simulink library "SUB_ECU_L4_MABX_HW_Interface_PTC_1571"  (R2018a)
settings: Solver=VariableStepAuto  StartTime=0.0  StopTime=10.0  RelTol=1e-3
PostLoadFcn:
  | , if any(exist('dsrtsu_mdlpostloadfcn', 'file') == [2, 3, 6]), try dsrtsu_mdlpostloadfcn('Execute', bdroot); catch fprintf('Error in PostLoadFcn (dsrtsu_mdlpostloadfcn) for model "%s":\n %s\n', bdroot, lasterr); end, end,
undefined symbols (not defined in the file or in its folder): CANR_PROPB_REAX_3_13_CHANNEL_APV, CANR_PROPB_REAX_4_13_CHANNEL_APV, CANR_PROPB_XPR_1_50_CHANNEL_APV, ENUM_CAN_RX_T, ENUM_CAN_TX_T, ENUM_REAX_OPERATION_MODE_T, ENUM_SIGNAL_HEALTH_T, ENUM_XBR_CONTROL_MODE_T, ENUM_XBR_EBI_MODE_T, ENUM_XBR_PASS_THROUGH_ACTIVE_T, ENUM_XBR_PRIORITY_T, ENUM_XPR_INHIBIT_PARK_MANUAL_T, ENUM_XPR_INHIBIT_UNPARK_MANUAL_T, ENUM_XPR_PARK_MANUAL_T, ENUM_XPR_UNPARK_MANUAL_T, IGNITION_RELAY_OVERRIDE_APV, INVERTER_RELAY_OVERRIDE_APV, MABX_RELAY_OVERRIDE_APV, PROPB_REAX_1_E4_DES_POS_SIG_SRC_APV, PROPB_REAX_1_E4_DESIRED_OPMODE_APV, PROPB_REAX_1_E4_DESIRED_POSITION_APV, ptc_matlab_lib, SENSOR_RELAY_OVERRIDE_APV, sfi, sfp
libraries: PTC_MBDS_LIB x163, rtican x81, simulink x41, EmE_MBD_Blockset x35, rti1401lib_dio_type4 x8, simulink_need_slupdate x7, $bdroot x5, rti1401lib_adc_type4 x2, rti1401lib_aio_type1 x1, rtitasklib x1
(part 5 of 27)

== system SUB_ECU_L4_MABX_HW_Interface_PTC_1571/DIGITAL_out/Shift Control ==
  In : Inport
  Bus Creator1 : BusCreator  Inputs=1
  Bus Selector : BusSelector  OutputSignals=INPUTS.DIO_Bus.ShiftControlDC
  Bus Selector1 : BusSelector  OutputSignals=INPUTS.CAN.ETC2_03.SPN524_TransSelectedGear,INPUTS.CAN.ETC2_03.SPN523_TransCurrentGear
  Compare To Zero : simulink/Logic and Bit Operations/Compare To Zero  relop===  OutDataTypeStr=boolean
  Compare To Zero1 : simulink/Logic and Bit Operations/Compare To Zero  relop===  OutDataTypeStr=boolean
  Constant : Constant  Value=.4
  Constant1 : Constant  Value=0.5
  Constant2 : Constant  Value=false
  F_ALLOW_ETC2_FOR_NEUTRAL_OUTPUT_APV : Constant  Value=true
  If_Then_Else : EmE_MBD_Blockset/Signal Routing/If_Then_Else
      settings: SourceProductName=PACCAR EmE MBD Blockset
  Logical Operator : Logic  OutDataTypeStr=boolean
  Logical Operator1 : Logic  OutDataTypeStr=boolean
  Logical Operator2 : Logic  Operator=OR  OutDataTypeStr=boolean
  Relational Operator : RelationalOperator  OutDataTypeStr=boolean  RndMeth=Nearest
  Relational Operator1 : RelationalOperator  Operator=<=  OutDataTypeStr=boolean  RndMeth=Nearest
  Out : Outport
  wires:
  Constant2/1 -> If_Then_Else/3
  F_ALLOW_ETC2_FOR_NEUTRAL_OUTPUT_APV/1 -> If_Then_Else/1
  If_Then_Else/1 -> Logical Operator2/2
  Logical Operator/1 -> Logical Operator2/1
  Logical Operator1/1 -> If_Then_Else/2
  Compare To Zero1/1 -> Logical Operator1/2
  Compare To Zero/1 -> Logical Operator1/1
  Bus Selector1/2 -> Compare To Zero1/1  "<SPN523_TransCurrentGear>"
  Bus Selector1/1 -> Compare To Zero/1  "<SPN524_TransSelectedGear>"
  Bus Selector/1 -> Relational Operator1/1, Relational Operator/1  "<ShiftControlDC>"
  Bus Creator1/1 -> Out/1
  Logical Operator2/1 -> Bus Creator1/1  "Neutral"
  Constant/1 -> Relational Operator/2
  Relational Operator1/1 -> Logical Operator/2
  Relational Operator/1 -> Logical Operator/1
  In/1 -> Bus Selector/1, Bus Selector1/1
  Constant1/1 -> Relational Operator1/2

== system SUB_ECU_L4_MABX_HW_Interface_PTC_1571/INPUTS_PTC_1571/Timer_Access ==
  IncrementTimer : Subsystem
  Rate Transition : RateTransition  Deterministic=off
  Timer Interrupt : rtitasklib/Timer Interrupt  DSProperties=struct('RTI',struct('Version',uint32(3),'BlockType',struct('isSLSource',uint8(1),'isSLSink',uint8(0),'isHWSource',uint8(0),'isHWSink',uint8(0),'isSetup',uint8(0),'isInline',uint8(1),'isNonInline',uint8(0),'isInterrupt',uint8(1),'isChannelwise',uint8(0)),'IOBoardType','INTLIB','UnitType','TMRINT','Identifier','TMRINT','DialogType','ML','BlockSet','NONE','SlaveProcessor','NONE','RelationId',struct('TH',struct('BlockId','TMRINT'))))  RTIBlockInterface=struct('OutputPortsActive',1,'OutputPortsWidth',int32(1),'FunctionCall',uint32(0),'OutputPortsName',{{[' ']}},'BlockDisplay',{{['DS1401 Board\nTimer B interrupt'],'center'}},'IconTransparency','on','InitLevel',3,'BlockName',struct('Token',{{['Timer Interrupt']}}),'DialogFcn','rtitasklibtmrintgui','SampleTime',{{-1}},'Options',{{'SS_OPTION_FORCE_NONINLINED_FCNCALL','SS_OPTION_ASYNCHRONOUS_INTERRUPT'}})  RTIBlockParameters=struct('ThPeriod',{{'0.01','OFF',[]}},'SampleTime',{{'-1','OFF',[]}},'ThTimerId',{{2,'OFF',[]}},'ThSrcSgnName',{{['Timer B interrupt'],'OFF',[]}},'ThBlk',{{['struct(''blkh'',[''SUB_ECU_L4_MABX_HW_Interface_PTC_1571/INPUTS_PTC_1571/Timer_Access/Timer Interrupt''],''srcId'',''TIMERB'',''srcSgnId'',''TIMERB'',''intervalTmrBlockId'',[],''srcSgnName'',[''Timer B interrupt''],''srcCpuId'','''',''isSrcCpu'',1,''isTargetCpu'',1,''srcOnMasterCpu'',1,''boardType'','''',''boardTypeNo'','''',''boardNo'',1,''intNo'',0,''subIntNo'',-1,''period'',''0.01'',''entryPoint'',''rti_TIMERB'',''blockName'',[''Timer Interrupt''],''taskNameDisplayExt'','''',''taskType'',''TMRINT'',''groupId'',''B'',''hookFcn'',''NULL'',''isTimerTaskSrc'',0,''service'',''S_PERIODIC_B'',''mpBlkId'','''',''taskPriorityPreConfig'',''none'',''taskPriority'',-1,''taskSortWeighting'',[],''taskSchedulingPolicy'',''FCFS'',''taskOvrPreConfig'',''none'',''taskOvrStrategy'',1,''taskOvrQueueSize'',1,''taskVisibility'',''on'',''taskGroupId'','''',''taskGroupDisplayOrder'',[],''serviceDynamicGen'',0,''disableCodeGen'',0,''boardBase'',''0'',''noBoardBase'','''')'],'OFF',[]}},'TLCFileName',{{'rtitasklibtmrint','OFF',[]}})  RTISFcnParameters=struct('ThBlk','struct','TLCFileName','char','SampleTime','double')  RTIBlockParaDefault=struct('ThPeriod',0.01,'SampleTime',-1,'ThTimerId',2,'ThSrcSgnName',['Timer B interrupt'],'ThBlk',['struct(''srcSgnId'', '''')'],'TLCFileName','rtitasklibtmrint')
  TimeStamp : Outport
  wires:
  Rate Transition/1 -> TimeStamp/1  "GLB_Absolute_Timestamp"
  IncrementTimer/1(Out1) -> Rate Transition/1
  Timer Interrupt/1 -> IncrementTimer/Trigger

== system SUB_ECU_L4_MABX_HW_Interface_PTC_1571/CAN_Out_PTC_1571/CAN_TX_1000ms/CAN_TX_AIR1_31 ==
  Channel : Inport  OutDataTypeStr=Enum: ENUM_CAN_TX_T
  Data : Inport  Port=2
  AND : PTC_MBDS_LIB/MBDS Standard Library/Basic Operations/Logic and Bit Operations/AND  BitwiseMode=on  Inputs=1  UseBitMask=on  BitMask=bin2dec('00000001')  OutDataTypeStr=Inherit: Inherit via back propagation  PTC_MBDS_BlockVersion=5.41  PTC_BlockType=PTC_MBDS_AND
      settings: AttributesFormatString=bitwise  SourceProductName=PACCAR Technical Center MBDS Library
  AND1 : PTC_MBDS_LIB/MBDS Standard Library/Basic Operations/Logic and Bit Operations/AND  BitwiseMode=on  Inputs=1  UseBitMask=on  BitMask=bin2dec('00000010')  OutDataTypeStr=Inherit: Inherit via back propagation  PTC_MBDS_BlockVersion=5.41  PTC_BlockType=PTC_MBDS_AND
      settings: AttributesFormatString=bitwise  SourceProductName=PACCAR Technical Center MBDS Library
  AND2 : PTC_MBDS_LIB/MBDS Standard Library/Basic Operations/Logic and Bit Operations/AND  BitwiseMode=on  Inputs=1  UseBitMask=on  BitMask=bin2dec('00000100')  OutDataTypeStr=Inherit: Inherit via back propagation  PTC_MBDS_BlockVersion=5.41  PTC_BlockType=PTC_MBDS_AND
      settings: AttributesFormatString=bitwise  SourceProductName=PACCAR Technical Center MBDS Library
  AND3 : PTC_MBDS_LIB/MBDS Standard Library/Basic Operations/Logic and Bit Operations/AND  BitwiseMode=on  Inputs=1  UseBitMask=on  BitMask=bin2dec('00001000')  OutDataTypeStr=Inherit: Inherit via back propagation  PTC_MBDS_BlockVersion=5.41  PTC_BlockType=PTC_MBDS_AND
      settings: AttributesFormatString=bitwise  SourceProductName=PACCAR Technical Center MBDS Library
  AND4 : PTC_MBDS_LIB/MBDS Standard Library/Basic Operations/Logic and Bit Operations/AND  BitwiseMode=on  Inputs=1  UseBitMask=on  BitMask=bin2dec('00010000')  OutDataTypeStr=Inherit: Inherit via back propagation  PTC_MBDS_BlockVersion=5.41  PTC_BlockType=PTC_MBDS_AND
      settings: AttributesFormatString=bitwise  SourceProductName=PACCAR Technical Center MBDS Library
  AND5 : PTC_MBDS_LIB/MBDS Standard Library/Basic Operations/Logic and Bit Operations/AND  BitwiseMode=on  Inputs=1  UseBitMask=on  BitMask=bin2dec('00100000')  OutDataTypeStr=Inherit: Inherit via back propagation  PTC_MBDS_BlockVersion=5.41  PTC_BlockType=PTC_MBDS_AND
      settings: AttributesFormatString=bitwise  SourceProductName=PACCAR Technical Center MBDS Library
  Data Type Conversion : DataTypeConversion  OutDataTypeStr=uint8  SaturateOnIntegerOverflow=on
  Data Type Conversion{2..7} (6 alike) : DataTypeConversion  OutDataTypeStr=boolean  SaturateOnIntegerOverflow=on
  "Shift_Arithmetic " : ArithShift  BitShiftNumber=1
  Shift_Arithmetic 1 : ArithShift  BitShiftNumber=2
  Shift_Arithmetic 2 : ArithShift  BitShiftNumber=3
  Shift_Arithmetic 3 : ArithShift  BitShiftNumber=4
  Shift_Arithmetic 4 : ArithShift  BitShiftNumber=5
  TX_CAN4 : Subsystem
  Terminator{,1..4} (5 alike) : Terminator
  wires:
  Shift_Arithmetic 4/1 -> Data Type Conversion7/1
  AND5/1 -> Shift_Arithmetic 4/1
  Shift_Arithmetic 3/1 -> Data Type Conversion6/1
  AND4/1 -> Shift_Arithmetic 3/1
  Shift_Arithmetic 2/1 -> Data Type Conversion5/1
  AND3/1 -> Shift_Arithmetic 2/1
  Shift_Arithmetic 1/1 -> Data Type Conversion4/1
  "Shift_Arithmetic "/1 -> Data Type Conversion3/1
  AND/1 -> Data Type Conversion2/1
  Data Type Conversion/1 -> AND2/1, AND3/1, AND5/1, AND4/1, AND1/1, AND/1
  Channel/1 -> Data Type Conversion/1
  AND2/1 -> Shift_Arithmetic 1/1
  AND1/1 -> "Shift_Arithmetic "/1
  Data/1 -> TX_CAN4/2(Data)
  Data Type Conversion2/1 -> Terminator/1
  Data Type Conversion3/1 -> Terminator1/1
  Data Type Conversion4/1 -> Terminator2/1
  Data Type Conversion6/1 -> Terminator3/1
  Data Type Conversion7/1 -> Terminator4/1
  Data Type Conversion5/1 -> TX_CAN4/1(Enable)

== system SUB_ECU_L4_MABX_HW_Interface_PTC_1571/CAN_Out_PTC_1571/CAN_TX_1000ms/CAN_TX_AMB_00 ==
  Channel : Inport  OutDataTypeStr=Enum: ENUM_CAN_TX_T
  Data : Inport  Port=2
  AND : PTC_MBDS_LIB/MBDS Standard Library/Basic Operations/Logic and Bit Operations/AND  BitwiseMode=on  Inputs=1  UseBitMask=on  BitMask=bin2dec('00000001')  OutDataTypeStr=Inherit: Inherit via back propagation  PTC_MBDS_BlockVersion=5.41  PTC_BlockType=PTC_MBDS_AND
      settings: AttributesFormatString=bitwise  SourceProductName=PACCAR Technical Center MBDS Library
  AND1 : PTC_MBDS_LIB/MBDS Standard Library/Basic Operations/Logic and Bit Operations/AND  BitwiseMode=on  Inputs=1  UseBitMask=on  BitMask=bin2dec('00000010')  OutDataTypeStr=Inherit: Inherit via back propagation  PTC_MBDS_BlockVersion=5.41  PTC_BlockType=PTC_MBDS_AND
      settings: AttributesFormatString=bitwise  SourceProductName=PACCAR Technical Center MBDS Library
  AND2 : PTC_MBDS_LIB/MBDS Standard Library/Basic Operations/Logic and Bit Operations/AND  BitwiseMode=on  Inputs=1  UseBitMask=on  BitMask=bin2dec('00000100')  OutDataTypeStr=Inherit: Inherit via back propagation  PTC_MBDS_BlockVersion=5.41  PTC_BlockType=PTC_MBDS_AND
      settings: AttributesFormatString=bitwise  SourceProductName=PACCAR Technical Center MBDS Library
  AND3 : PTC_MBDS_LIB/MBDS Standard Library/Basic Operations/Logic and Bit Operations/AND  BitwiseMode=on  Inputs=1  UseBitMask=on  BitMask=bin2dec('00001000')  OutDataTypeStr=Inherit: Inherit via back propagation  PTC_MBDS_BlockVersion=5.41  PTC_BlockType=PTC_MBDS_AND
      settings: AttributesFormatString=bitwise  SourceProductName=PACCAR Technical Center MBDS Library
  AND4 : PTC_MBDS_LIB/MBDS Standard Library/Basic Operations/Logic and Bit Operations/AND  BitwiseMode=on  Inputs=1  UseBitMask=on  BitMask=bin2dec('00010000')  OutDataTypeStr=Inherit: Inherit via back propagation  PTC_MBDS_BlockVersion=5.41  PTC_BlockType=PTC_MBDS_AND
      settings: AttributesFormatString=bitwise  SourceProductName=PACCAR Technical Center MBDS Library
  AND5 : PTC_MBDS_LIB/MBDS Standard Library/Basic Operations/Logic and Bit Operations/AND  BitwiseMode=on  Inputs=1  UseBitMask=on  BitMask=bin2dec('00100000')  OutDataTypeStr=Inherit: Inherit via back propagation  PTC_MBDS_BlockVersion=5.41  PTC_BlockType=PTC_MBDS_AND
      settings: AttributesFormatString=bitwise  SourceProductName=PACCAR Technical Center MBDS Library
  Data Type Conversion : DataTypeConversion  OutDataTypeStr=uint8  SaturateOnIntegerOverflow=on
  Data Type Conversion{2..7} (6 alike) : DataTypeConversion  OutDataTypeStr=boolean  SaturateOnIntegerOverflow=on
  "Shift_Arithmetic " : ArithShift  BitShiftNumber=1
  Shift_Arithmetic 1 : ArithShift  BitShiftNumber=2
  Shift_Arithmetic 2 : ArithShift  BitShiftNumber=3
  Shift_Arithmetic 3 : ArithShift  BitShiftNumber=4
  Shift_Arithmetic 4 : ArithShift  BitShiftNumber=5
  TX_CAN4 : Subsystem
  Terminator{,1..4} (5 alike) : Terminator
  wires:
  Data Type Conversion5/1 -> TX_CAN4/1(Enable)
  Data Type Conversion7/1 -> Terminator4/1
  Data Type Conversion6/1 -> Terminator3/1
  Data Type Conversion4/1 -> Terminator2/1
  Data Type Conversion3/1 -> Terminator1/1
  Data Type Conversion2/1 -> Terminator/1
  Data/1 -> TX_CAN4/2(Data)
  AND1/1 -> "Shift_Arithmetic "/1
  AND2/1 -> Shift_Arithmetic 1/1
  Channel/1 -> Data Type Conversion/1
  Data Type Conversion/1 -> AND/1, AND1/1, AND4/1, AND5/1, AND3/1, AND2/1
  AND/1 -> Data Type Conversion2/1
  "Shift_Arithmetic "/1 -> Data Type Conversion3/1
  Shift_Arithmetic 1/1 -> Data Type Conversion4/1
  AND3/1 -> Shift_Arithmetic 2/1
  Shift_Arithmetic 2/1 -> Data Type Conversion5/1
  AND4/1 -> Shift_Arithmetic 3/1
  Shift_Arithmetic 3/1 -> Data Type Conversion6/1
  AND5/1 -> Shift_Arithmetic 4/1
  Shift_Arithmetic 4/1 -> Data Type Conversion7/1

== system SUB_ECU_L4_MABX_HW_Interface_PTC_1571/CAN_Out_PTC_1571/CAN_TX_100ms/CAN_TX_CCVS1_00 ==
  Data : Inport
  Enable_TX_CCVS1_00 : Constant  Value=boolean(1)
  TX_CAN4 : Subsystem
  TX_CAN5 : Subsystem
  wires:
  Enable_TX_CCVS1_00/1 -> TX_CAN4/1(Enable), TX_CAN5/1(Enable)
  Data/1 -> TX_CAN4/2(Data), TX_CAN5/2(Data)

== system SUB_ECU_L4_MABX_HW_Interface_PTC_1571/CAN_Out_PTC_1571/CAN_TX_100ms/CAN_TX_CCVS1_31 ==
  Data : Inport
  Enable_TX_CCVS1_31 : Constant  Value=boolean(1)
  TX_CAN3 : Subsystem
  wires:
  Data/1 -> TX_CAN3/2(Data)
  Enable_TX_CCVS1_31/1 -> TX_CAN3/1(Enable)

== system SUB_ECU_L4_MABX_HW_Interface_PTC_1571/CAN_Out_PTC_1571/CAN_TX_100ms/CAN_TX_EBC2_0B ==
  Data : Inport
  Enable_TX_EBC2_0B : Constant  Value=boolean(1)
  TX_CAN3 : Subsystem
  wires:
  Enable_TX_EBC2_0B/1 -> TX_CAN3/1(Enable)
  Data/1 -> TX_CAN3/2(Data)

== system SUB_ECU_L4_MABX_HW_Interface_PTC_1571/CAN_Out_PTC_1571/CAN_TX_100ms/CAN_TX_ETC2_03 ==
  Data : Inport
  Enable_TX_ETC2_03 : Constant  Value=boolean(1)
  TX_CAN3 : Subsystem
  wires:
  Data/1 -> TX_CAN3/2(Data)
  Enable_TX_ETC2_03/1 -> TX_CAN3/1(Enable)

== system SUB_ECU_L4_MABX_HW_Interface_PTC_1571/CAN_Out_PTC_1571/CAN_TX_100ms/CAN_TX_PROPB_REAX_5_E4 ==
  enable : Inport
  RawData : Inport  Port=2  OutDataTypeStr=uint8
  Bus Selector : BusSelector  OutputSignals=INPUTS.CAN.CANenable.EnablePropB_ReAX_CAN1,INPUTS.CAN.CANenable.EnablePropB_ReAX_CAN2
  Data Type Conversion1 : DataTypeConversion  SaturateOnIntegerOverflow=on
  TX_CAN1 : Subsystem
  TX_CAN2 : Subsystem
  wires:
  Bus Selector/1 -> TX_CAN1/1(Enable)  "<EnablePropB_ReAX_CAN1>"
  Data Type Conversion1/1 -> TX_CAN2/2(RawData), TX_CAN1/2(RawData)
  RawData/1 -> Data Type Conversion1/1
  enable/1 -> Bus Selector/1
  Bus Selector/2 -> TX_CAN2/1(Enable)  "<EnablePropB_ReAX_CAN2>"

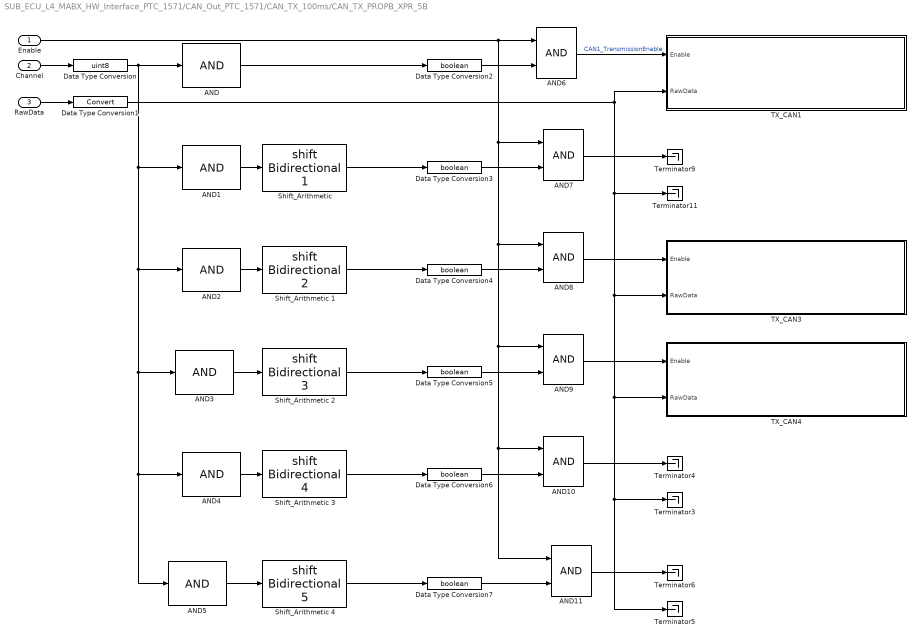
== system SUB_ECU_L4_MABX_HW_Interface_PTC_1571/CAN_Out_PTC_1571/CAN_TX_100ms/CAN_TX_PROPB_XPR_5B ==
  Enable : Inport
  Channel : Inport  Port=2  OutDataTypeStr=Enum: ENUM_CAN_TX_T
  RawData : Inport  Port=3  OutDataTypeStr=uint8
  AND : PTC_MBDS_LIB/MBDS Standard Library/Basic Operations/Logic and Bit Operations/AND  BitwiseMode=on  Inputs=1  UseBitMask=on  BitMask=bin2dec('00000001')  OutDataTypeStr=Inherit: Inherit via back propagation  PTC_MBDS_BlockVersion=5.41  PTC_BlockType=PTC_MBDS_AND
      settings: AttributesFormatString=bitwise  SourceProductName=PACCAR Technical Center MBDS Library
  AND1 : PTC_MBDS_LIB/MBDS Standard Library/Basic Operations/Logic and Bit Operations/AND  BitwiseMode=on  Inputs=1  UseBitMask=on  BitMask=bin2dec('00000010')  OutDataTypeStr=Inherit: Inherit via back propagation  PTC_MBDS_BlockVersion=5.41  PTC_BlockType=PTC_MBDS_AND
      settings: AttributesFormatString=bitwise  SourceProductName=PACCAR Technical Center MBDS Library
  AND{6..11} (6 alike) : PTC_MBDS_LIB/MBDS Standard Library/Basic Operations/Logic and Bit Operations/AND  BitwiseMode=off  Inputs=2  UseBitMask=off  BitMask='A7'  OutDataTypeStr=Inherit: Inherit via back propagation  PTC_MBDS_BlockVersion=5.41  PTC_BlockType=PTC_MBDS_AND
      settings: SourceProductName=PACCAR Technical Center MBDS Library
  AND2 : PTC_MBDS_LIB/MBDS Standard Library/Basic Operations/Logic and Bit Operations/AND  BitwiseMode=on  Inputs=1  UseBitMask=on  BitMask=bin2dec('00000100')  OutDataTypeStr=Inherit: Inherit via back propagation  PTC_MBDS_BlockVersion=5.41  PTC_BlockType=PTC_MBDS_AND
      settings: AttributesFormatString=bitwise  SourceProductName=PACCAR Technical Center MBDS Library
  AND3 : PTC_MBDS_LIB/MBDS Standard Library/Basic Operations/Logic and Bit Operations/AND  BitwiseMode=on  Inputs=1  UseBitMask=on  BitMask=bin2dec('00001000')  OutDataTypeStr=Inherit: Inherit via back propagation  PTC_MBDS_BlockVersion=5.41  PTC_BlockType=PTC_MBDS_AND
      settings: AttributesFormatString=bitwise  SourceProductName=PACCAR Technical Center MBDS Library
  AND4 : PTC_MBDS_LIB/MBDS Standard Library/Basic Operations/Logic and Bit Operations/AND  BitwiseMode=on  Inputs=1  UseBitMask=on  BitMask=bin2dec('00010000')  OutDataTypeStr=Inherit: Inherit via back propagation  PTC_MBDS_BlockVersion=5.41  PTC_BlockType=PTC_MBDS_AND
      settings: AttributesFormatString=bitwise  SourceProductName=PACCAR Technical Center MBDS Library
  AND5 : PTC_MBDS_LIB/MBDS Standard Library/Basic Operations/Logic and Bit Operations/AND  BitwiseMode=on  Inputs=1  UseBitMask=on  BitMask=bin2dec('00100000')  OutDataTypeStr=Inherit: Inherit via back propagation  PTC_MBDS_BlockVersion=5.41  PTC_BlockType=PTC_MBDS_AND
      settings: AttributesFormatString=bitwise  SourceProductName=PACCAR Technical Center MBDS Library
  Data Type Conversion : DataTypeConversion  OutDataTypeStr=uint8  SaturateOnIntegerOverflow=on
  Data Type Conversion1 : DataTypeConversion  SaturateOnIntegerOverflow=on
  Data Type Conversion{2..7} (6 alike) : DataTypeConversion  OutDataTypeStr=boolean  SaturateOnIntegerOverflow=on
  "Shift_Arithmetic " : ArithShift  BitShiftNumber=1
  Shift_Arithmetic 1 : ArithShift  BitShiftNumber=2
  Shift_Arithmetic 2 : ArithShift  BitShiftNumber=3
  Shift_Arithmetic 3 : ArithShift  BitShiftNumber=4
  Shift_Arithmetic 4 : ArithShift  BitShiftNumber=5
  TX_CAN1 : Subsystem
  TX_CAN3 : Subsystem
  TX_CAN4 : Subsystem
  Terminator{3..6,9,11} (6 alike) : Terminator
  wires:
  AND6/1 -> TX_CAN1/1(Enable)  "CAN1_TransmissionEnable"
  AND7/1 -> Terminator9/1
  AND8/1 -> TX_CAN3/1(Enable)
  AND9/1 -> TX_CAN4/1(Enable)
  AND10/1 -> Terminator4/1
  AND11/1 -> Terminator6/1
  Enable/1 -> AND6/1, AND7/1, AND8/1, AND9/1, AND10/1, AND11/1
  Data Type Conversion7/1 -> AND11/2
  Data Type Conversion6/1 -> AND10/2
  Data Type Conversion5/1 -> AND9/2
  Data Type Conversion4/1 -> AND8/2
  Data Type Conversion3/1 -> AND7/2
  Data Type Conversion2/1 -> AND6/2
  Data Type Conversion1/1 -> Terminator11/1, TX_CAN3/2(RawData), Terminator5/1, Terminator3/1, TX_CAN4/2(RawData), TX_CAN1/2(RawData)
  AND1/1 -> "Shift_Arithmetic "/1
  AND2/1 -> Shift_Arithmetic 1/1
  Channel/1 -> Data Type Conversion/1
  Data Type Conversion/1 -> AND/1, AND1/1, AND4/1, AND5/1, AND3/1, AND2/1
  RawData/1 -> Data Type Conversion1/1
  AND/1 -> Data Type Conversion2/1
  "Shift_Arithmetic "/1 -> Data Type Conversion3/1
  Shift_Arithmetic 1/1 -> Data Type Conversion4/1
  AND3/1 -> Shift_Arithmetic 2/1
  Shift_Arithmetic 2/1 -> Data Type Conversion5/1
  AND4/1 -> Shift_Arithmetic 3/1
  Shift_Arithmetic 3/1 -> Data Type Conversion6/1
  AND5/1 -> Shift_Arithmetic 4/1
  Shift_Arithmetic 4/1 -> Data Type Conversion7/1

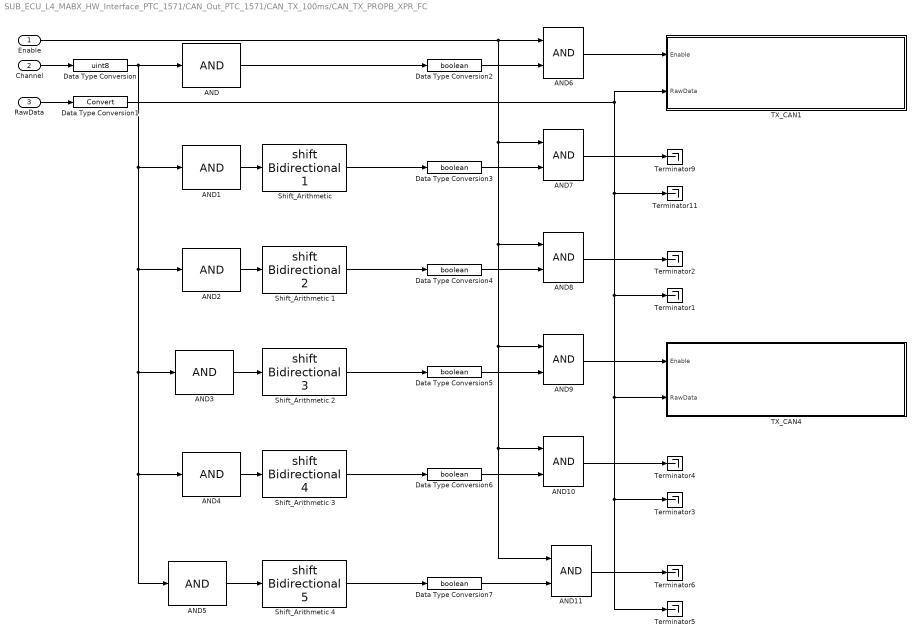
== system SUB_ECU_L4_MABX_HW_Interface_PTC_1571/CAN_Out_PTC_1571/CAN_TX_100ms/CAN_TX_PROPB_XPR_FC ==
  Enable : Inport
  Channel : Inport  Port=2  OutDataTypeStr=Enum: ENUM_CAN_TX_T
  RawData : Inport  Port=3  OutDataTypeStr=uint8
  AND : PTC_MBDS_LIB/MBDS Standard Library/Basic Operations/Logic and Bit Operations/AND  BitwiseMode=on  Inputs=1  UseBitMask=on  BitMask=bin2dec('00000001')  OutDataTypeStr=Inherit: Inherit via back propagation  PTC_MBDS_BlockVersion=5.41  PTC_BlockType=PTC_MBDS_AND
      settings: AttributesFormatString=bitwise  SourceProductName=PACCAR Technical Center MBDS Library
  AND1 : PTC_MBDS_LIB/MBDS Standard Library/Basic Operations/Logic and Bit Operations/AND  BitwiseMode=on  Inputs=1  UseBitMask=on  BitMask=bin2dec('00000010')  OutDataTypeStr=Inherit: Inherit via back propagation  PTC_MBDS_BlockVersion=5.41  PTC_BlockType=PTC_MBDS_AND
      settings: AttributesFormatString=bitwise  SourceProductName=PACCAR Technical Center MBDS Library
  AND{6..11} (6 alike) : PTC_MBDS_LIB/MBDS Standard Library/Basic Operations/Logic and Bit Operations/AND  BitwiseMode=off  Inputs=2  UseBitMask=off  BitMask='A7'  OutDataTypeStr=Inherit: Inherit via back propagation  PTC_MBDS_BlockVersion=5.41  PTC_BlockType=PTC_MBDS_AND
      settings: SourceProductName=PACCAR Technical Center MBDS Library
  AND2 : PTC_MBDS_LIB/MBDS Standard Library/Basic Operations/Logic and Bit Operations/AND  BitwiseMode=on  Inputs=1  UseBitMask=on  BitMask=bin2dec('00000100')  OutDataTypeStr=Inherit: Inherit via back propagation  PTC_MBDS_BlockVersion=5.41  PTC_BlockType=PTC_MBDS_AND
      settings: AttributesFormatString=bitwise  SourceProductName=PACCAR Technical Center MBDS Library
  AND3 : PTC_MBDS_LIB/MBDS Standard Library/Basic Operations/Logic and Bit Operations/AND  BitwiseMode=on  Inputs=1  UseBitMask=on  BitMask=bin2dec('00001000')  OutDataTypeStr=Inherit: Inherit via back propagation  PTC_MBDS_BlockVersion=5.41  PTC_BlockType=PTC_MBDS_AND
      settings: AttributesFormatString=bitwise  SourceProductName=PACCAR Technical Center MBDS Library
  AND4 : PTC_MBDS_LIB/MBDS Standard Library/Basic Operations/Logic and Bit Operations/AND  BitwiseMode=on  Inputs=1  UseBitMask=on  BitMask=bin2dec('00010000')  OutDataTypeStr=Inherit: Inherit via back propagation  PTC_MBDS_BlockVersion=5.41  PTC_BlockType=PTC_MBDS_AND
      settings: AttributesFormatString=bitwise  SourceProductName=PACCAR Technical Center MBDS Library
  AND5 : PTC_MBDS_LIB/MBDS Standard Library/Basic Operations/Logic and Bit Operations/AND  BitwiseMode=on  Inputs=1  UseBitMask=on  BitMask=bin2dec('00100000')  OutDataTypeStr=Inherit: Inherit via back propagation  PTC_MBDS_BlockVersion=5.41  PTC_BlockType=PTC_MBDS_AND
      settings: AttributesFormatString=bitwise  SourceProductName=PACCAR Technical Center MBDS Library
  Data Type Conversion : DataTypeConversion  OutDataTypeStr=uint8  SaturateOnIntegerOverflow=on
  Data Type Conversion1 : DataTypeConversion  SaturateOnIntegerOverflow=on
  Data Type Conversion{2..7} (6 alike) : DataTypeConversion  OutDataTypeStr=boolean  SaturateOnIntegerOverflow=on
  "Shift_Arithmetic " : ArithShift  BitShiftNumber=1
  Shift_Arithmetic 1 : ArithShift  BitShiftNumber=2
  Shift_Arithmetic 2 : ArithShift  BitShiftNumber=3
  Shift_Arithmetic 3 : ArithShift  BitShiftNumber=4
  Shift_Arithmetic 4 : ArithShift  BitShiftNumber=5
  TX_CAN1 : Subsystem
  TX_CAN4 : Subsystem
  Terminator{1..6,9,11} (8 alike) : Terminator
  wires:
  Shift_Arithmetic 4/1 -> Data Type Conversion7/1
  AND5/1 -> Shift_Arithmetic 4/1
  Shift_Arithmetic 3/1 -> Data Type Conversion6/1
  AND4/1 -> Shift_Arithmetic 3/1
  Shift_Arithmetic 2/1 -> Data Type Conversion5/1
  AND3/1 -> Shift_Arithmetic 2/1
  Shift_Arithmetic 1/1 -> Data Type Conversion4/1
  "Shift_Arithmetic "/1 -> Data Type Conversion3/1
  AND/1 -> Data Type Conversion2/1
  RawData/1 -> Data Type Conversion1/1
  Data Type Conversion/1 -> AND2/1, AND3/1, AND5/1, AND4/1, AND1/1, AND/1
  Channel/1 -> Data Type Conversion/1
  AND2/1 -> Shift_Arithmetic 1/1
  AND1/1 -> "Shift_Arithmetic "/1
  Data Type Conversion1/1 -> TX_CAN1/2(RawData), Terminator11/1, Terminator1/1, TX_CAN4/2(RawData), Terminator5/1, Terminator3/1
  Data Type Conversion2/1 -> AND6/2
  Data Type Conversion3/1 -> AND7/2
  Data Type Conversion4/1 -> AND8/2
  Data Type Conversion5/1 -> AND9/2
  Data Type Conversion6/1 -> AND10/2
  Data Type Conversion7/1 -> AND11/2
  Enable/1 -> AND11/1, AND10/1, AND9/1, AND8/1, AND7/1, AND6/1
  AND11/1 -> Terminator6/1
  AND10/1 -> Terminator4/1
  AND9/1 -> TX_CAN4/1(Enable)
  AND8/1 -> Terminator2/1
  AND7/1 -> Terminator9/1
  AND6/1 -> TX_CAN1/1(Enable)

== system SUB_ECU_L4_MABX_HW_Interface_PTC_1571/CAN_Out_PTC_1571/CAN_TX_100ms/COGSRapidUpdate ==
  Enable : Inport
  Data : Inport  Port=2
  Data Type Conversion2 : DataTypeConversion  OutDataTypeStr=boolean  SaturateOnIntegerOverflow=on
  TX : Subsystem
  wires:
  Enable/1 -> Data Type Conversion2/1
  Data/1 -> TX/2(Data)
  Data Type Conversion2/1 -> TX/1(Enable)

== system SUB_ECU_L4_MABX_HW_Interface_PTC_1571/CAN_Out_PTC_1571/CAN_TX_100ms/EBC1_8B ==
  Enable : Inport
  Data : Inport  Port=2
  Data Type Conversion2 : DataTypeConversion  OutDataTypeStr=boolean  SaturateOnIntegerOverflow=on
  TX_EBC1_8B : Subsystem
  wires:
  Data Type Conversion2/1 -> TX_EBC1_8B/1(Enable)
  Data/1 -> TX_EBC1_8B/2(Data)
  Enable/1 -> Data Type Conversion2/1

== system SUB_ECU_L4_MABX_HW_Interface_PTC_1571/CAN_Out_PTC_1571/CAN_TX_100ms/EffortsValue ==
  Constant : Constant  Value=int16(512)
  EffortsValue : Outport
  wires:
  Constant/1 -> EffortsValue/1

== system SUB_ECU_L4_MABX_HW_Interface_PTC_1571/CAN_Out_PTC_1571/CAN_TX_100ms/Encode_PropB_REAX_5 ==
  EffortsValue : Inport
  AND : PTC_MBDS_LIB/MBDS Standard Library/Basic Operations/Logic and Bit Operations/AND  BitwiseMode=on  Inputs=1  UseBitMask=on  BitMask='00FF'  OutDataTypeStr=uint8  PTC_MBDS_BlockVersion=5.41  PTC_BlockType=PTC_MBDS_AND
      settings: AttributesFormatString=bitwise  SourceProductName=PACCAR Technical Center MBDS Library
  AND1 : PTC_MBDS_LIB/MBDS Standard Library/Basic Operations/Logic and Bit Operations/AND  BitwiseMode=on  Inputs=1  UseBitMask=on  BitMask='FF00'  OutDataTypeStr=uint16  PTC_MBDS_BlockVersion=5.41  PTC_BlockType=PTC_MBDS_AND
      settings: AttributesFormatString=bitwise  SourceProductName=PACCAR Technical Center MBDS Library
  Constant : Constant  Value=uint8(hex2dec('FF'))
  Data Type Conversion : DataTypeConversion  OutDataTypeStr=int16  SaturateOnIntegerOverflow=on
  Data Type Conversion1 : DataTypeConversion  OutDataTypeStr=uint16  ConvertRealWorld=Stored Integer (SI)
  Data Type Conversion2 : DataTypeConversion  OutDataTypeStr=uint8  SaturateOnIntegerOverflow=on
  Mux : Mux  Inputs=8
  "Shift_Arithmetic " : ArithShift  BitShiftNumber=8
  Data : Outport
  wires:
  Mux/1 -> Data/1
  Constant/1 -> Mux/1, Mux/2, Mux/4, Mux/5, Mux/6, Mux/3
  Data Type Conversion2/1 -> Mux/8
  AND/1 -> Mux/7
  "Shift_Arithmetic "/1 -> Data Type Conversion2/1
  AND1/1 -> "Shift_Arithmetic "/1
  Data Type Conversion1/1 -> AND/1, AND1/1
  Data Type Conversion/1 -> Data Type Conversion1/1
  EffortsValue/1 -> Data Type Conversion/1

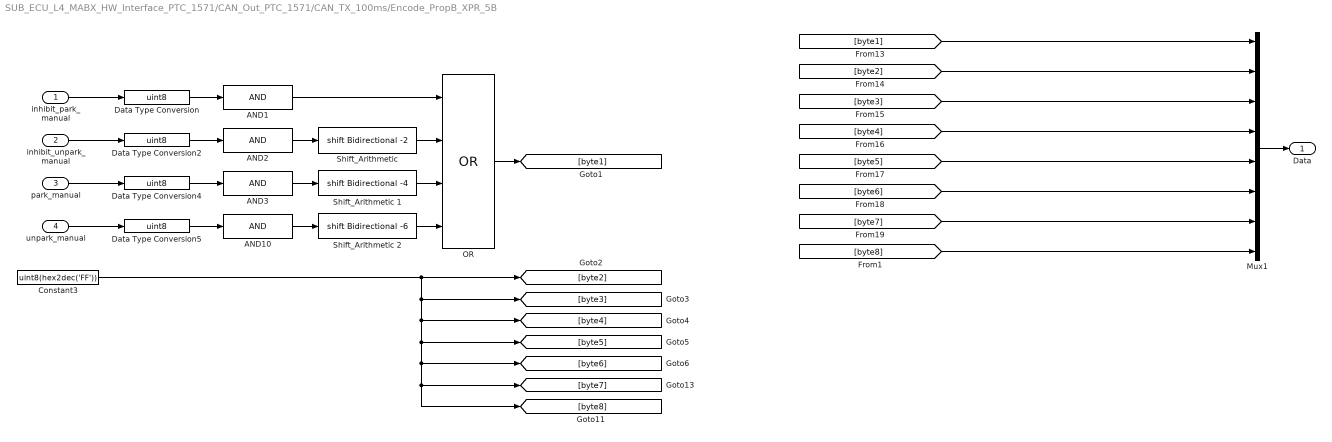
== system SUB_ECU_L4_MABX_HW_Interface_PTC_1571/CAN_Out_PTC_1571/CAN_TX_100ms/Encode_PropB_XPR_5B ==
  inhibit_park_manual : Inport
  inhibit_unpark_manual : Inport  Port=2
  park_manual : Inport  Port=3
  unpark_manual : Inport  Port=4
  AND{1..3,10} (4 alike) : PTC_MBDS_LIB/MBDS Standard Library/Basic Operations/Logic and Bit Operations/AND  BitwiseMode=on  Inputs=1  UseBitMask=on  BitMask=bin2dec('00000011')  OutDataTypeStr=uint8  PTC_MBDS_BlockVersion=5.41  PTC_BlockType=PTC_MBDS_AND
      settings: AttributesFormatString=bitwise  SourceProductName=PACCAR Technical Center MBDS Library
  Constant3 : Constant  Value=uint8(hex2dec('FF'))
  Data Type Conversion{,2,4..5} (4 alike) : DataTypeConversion  OutMin=0  OutMax=3  OutDataTypeStr=uint8  SaturateOnIntegerOverflow=on
  Mux1 : Mux  Inputs=8
  OR : PTC_MBDS_LIB/MBDS Standard Library/Basic Operations/Logic and Bit Operations/OR  BitwiseMode=on  Inputs=4  UseBitMask=off  BitMask='A7'  OutDataTypeStr=uint8  PTC_MBDS_BlockVersion=5.41  PTC_BlockType=PTC_MBDS_OR
      settings: AttributesFormatString=bitwise  SourceProductName=PACCAR Technical Center MBDS Library
  "Shift_Arithmetic " : ArithShift  BitShiftNumber=-2
  Shift_Arithmetic 1 : ArithShift  BitShiftNumber=-4
  Shift_Arithmetic 2 : ArithShift  BitShiftNumber=-6
  Data : Outport
  wires:
  [byte8] -> Mux1/8
  AND10/1 -> Shift_Arithmetic 2/1
  AND3/1 -> Shift_Arithmetic 1/1
  AND2/1 -> "Shift_Arithmetic "/1
  AND1/1 -> OR/1
  Data Type Conversion5/1 -> AND10/1
  Data Type Conversion4/1 -> AND3/1
  Data Type Conversion2/1 -> AND2/1
  OR/1 -> [byte1]
  Shift_Arithmetic 2/1 -> OR/4
  Shift_Arithmetic 1/1 -> OR/3
  Data Type Conversion/1 -> AND1/1
  "Shift_Arithmetic "/1 -> OR/2
  unpark_manual/1 -> Data Type Conversion5/1
  park_manual/1 -> Data Type Conversion4/1
  inhibit_unpark_manual/1 -> Data Type Conversion2/1
  inhibit_park_manual/1 -> Data Type Conversion/1
  [byte6] -> Mux1/6
  [byte5] -> Mux1/5
  [byte4] -> Mux1/4
  [byte3] -> Mux1/3
  [byte2] -> Mux1/2
  [byte1] -> Mux1/1
  Constant3/1 -> [byte2], [byte3], [byte4], [byte5], [byte6], [byte7], [byte8]
  Mux1/1 -> Data/1
  [byte7] -> Mux1/7

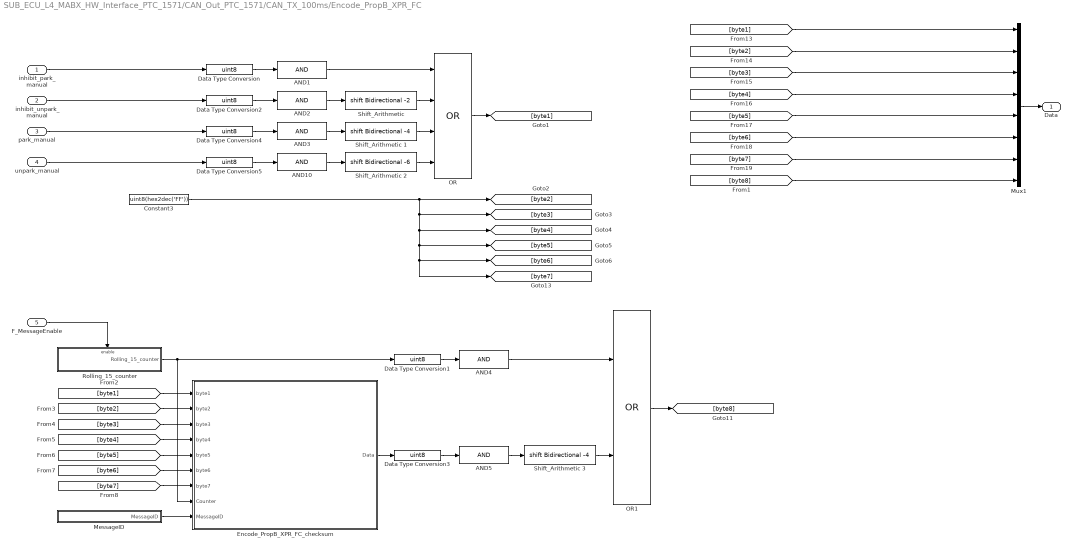
== system SUB_ECU_L4_MABX_HW_Interface_PTC_1571/CAN_Out_PTC_1571/CAN_TX_100ms/Encode_PropB_XPR_FC ==
  inhibit_park_manual : Inport
  inhibit_unpark_manual : Inport  Port=2
  park_manual : Inport  Port=3
  unpark_manual : Inport  Port=4
  F_MessageEnable : Inport  Port=5
  AND{1..3,10} (4 alike) : PTC_MBDS_LIB/MBDS Standard Library/Basic Operations/Logic and Bit Operations/AND  BitwiseMode=on  Inputs=1  UseBitMask=on  BitMask=bin2dec('00000011')  OutDataTypeStr=uint8  PTC_MBDS_BlockVersion=5.41  PTC_BlockType=PTC_MBDS_AND
      settings: AttributesFormatString=bitwise  SourceProductName=PACCAR Technical Center MBDS Library
  AND4 : PTC_MBDS_LIB/MBDS Standard Library/Basic Operations/Logic and Bit Operations/AND  BitwiseMode=on  Inputs=1  UseBitMask=on  BitMask=bin2dec('00001111')  OutDataTypeStr=uint8  PTC_MBDS_BlockVersion=5.41  PTC_BlockType=PTC_MBDS_AND
      settings: AttributesFormatString=bitwise  SourceProductName=PACCAR Technical Center MBDS Library
  AND5 : PTC_MBDS_LIB/MBDS Standard Library/Basic Operations/Logic and Bit Operations/AND  BitwiseMode=on  Inputs=1  UseBitMask=on  BitMask=bin2dec('00001111')  OutDataTypeStr=uint8  PTC_MBDS_BlockVersion=5.41  PTC_BlockType=PTC_MBDS_AND
      settings: AttributesFormatString=bitwise  SourceProductName=PACCAR Technical Center MBDS Library
  Constant3 : Constant  Value=uint8(hex2dec('FF'))
  Data Type Conversion{,1..5} (6 alike) : DataTypeConversion  OutMin=0  OutMax=3  OutDataTypeStr=uint8  SaturateOnIntegerOverflow=on
  Encode_PropB_XPR_FC_checksum : Subsystem
  MessageID : Subsystem
  Mux1 : Mux  Inputs=8
  OR : PTC_MBDS_LIB/MBDS Standard Library/Basic Operations/Logic and Bit Operations/OR  BitwiseMode=on  Inputs=4  UseBitMask=off  BitMask='A7'  OutDataTypeStr=uint8  PTC_MBDS_BlockVersion=5.41  PTC_BlockType=PTC_MBDS_OR
      settings: AttributesFormatString=bitwise  SourceProductName=PACCAR Technical Center MBDS Library
  OR1 : PTC_MBDS_LIB/MBDS Standard Library/Basic Operations/Logic and Bit Operations/OR  BitwiseMode=on  Inputs=2  UseBitMask=off  BitMask='A7'  OutDataTypeStr=uint8  PTC_MBDS_BlockVersion=5.41  PTC_BlockType=PTC_MBDS_OR
      settings: AttributesFormatString=bitwise  SourceProductName=PACCAR Technical Center MBDS Library
  Rolling_15_counter : Subsystem
  "Shift_Arithmetic " : ArithShift  BitShiftNumber=-2
  Shift_Arithmetic 1 : ArithShift  BitShiftNumber=-4
  Shift_Arithmetic 2 : ArithShift  BitShiftNumber=-6
  Shift_Arithmetic 3 : ArithShift  BitShiftNumber=-4
  Data : Outport
  wires:
  [byte8] -> Mux1/8
  AND10/1 -> Shift_Arithmetic 2/1
  AND3/1 -> Shift_Arithmetic 1/1
  AND2/1 -> "Shift_Arithmetic "/1
  AND1/1 -> OR/1
  Data Type Conversion5/1 -> AND10/1
  Data Type Conversion4/1 -> AND3/1
  Data Type Conversion2/1 -> AND2/1
  OR/1 -> [byte1]
  Shift_Arithmetic 2/1 -> OR/4
  Shift_Arithmetic 1/1 -> OR/3
  Data Type Conversion/1 -> AND1/1
  "Shift_Arithmetic "/1 -> OR/2
  unpark_manual/1 -> Data Type Conversion5/1
  park_manual/1 -> Data Type Conversion4/1
  inhibit_unpark_manual/1 -> Data Type Conversion2/1
  inhibit_park_manual/1 -> Data Type Conversion/1
  [byte6] -> Mux1/6
  [byte5] -> Mux1/5
  [byte4] -> Mux1/4
  [byte3] -> Mux1/3
  [byte2] -> Mux1/2
  [byte1] -> Mux1/1
  Constant3/1 -> [byte2], [byte3], [byte4], [byte5], [byte6], [byte7]
  Mux1/1 -> Data/1
  [byte7] -> Mux1/7
  Rolling_15_counter/1(Rolling_15_counter) -> Data Type Conversion1/1, Encode_PropB_XPR_FC_checksum/8(Counter)
  MessageID/1(MessageID) -> Encode_PropB_XPR_FC_checksum/9(MessageID)
  Data Type Conversion1/1 -> AND4/1
  Data Type Conversion3/1 -> AND5/1
  Encode_PropB_XPR_FC_checksum/1(Data) -> Data Type Conversion3/1
  AND5/1 -> Shift_Arithmetic 3/1
  AND4/1 -> OR1/1
  Shift_Arithmetic 3/1 -> OR1/2
  OR1/1 -> [byte8]
  [byte7] -> Encode_PropB_XPR_FC_checksum/7(byte7)
  [byte6] -> Encode_PropB_XPR_FC_checksum/6(byte6)
  [byte5] -> Encode_PropB_XPR_FC_checksum/5(byte5)
  [byte4] -> Encode_PropB_XPR_FC_checksum/4(byte4)
  [byte3] -> Encode_PropB_XPR_FC_checksum/3(byte3)
  [byte2] -> Encode_PropB_XPR_FC_checksum/2(byte2)
  [byte1] -> Encode_PropB_XPR_FC_checksum/1(byte1)
  F_MessageEnable/1 -> Rolling_15_counter/Enable

== system SUB_ECU_L4_MABX_HW_Interface_PTC_1571/CAN_Out_PTC_1571/CAN_TX_100ms/POSRapidUpdate ==
  Enable : Inport
  Data : Inport  Port=2
  Data Type Conversion2 : DataTypeConversion  OutDataTypeStr=boolean  SaturateOnIntegerOverflow=on
  TX : Subsystem
  wires:
  Data Type Conversion2/1 -> TX/1(Enable)
  Data/1 -> TX/2(Data)
  Enable/1 -> Data Type Conversion2/1

== system SUB_ECU_L4_MABX_HW_Interface_PTC_1571/CAN_Out_PTC_1571/CAN_TX_10ms/CAN_TX_ACCS_E4 ==
  Channel : Inport  OutDataTypeStr=Enum: ENUM_CAN_TX_T
  Data : Inport  Port=2
  AND : PTC_MBDS_LIB/MBDS Standard Library/Basic Operations/Logic and Bit Operations/AND  BitwiseMode=on  Inputs=1  UseBitMask=on  BitMask=bin2dec('00000001')  OutDataTypeStr=Inherit: Inherit via back propagation  PTC_MBDS_BlockVersion=5.41  PTC_BlockType=PTC_MBDS_AND
      settings: AttributesFormatString=bitwise  SourceProductName=PACCAR Technical Center MBDS Library
  AND1 : PTC_MBDS_LIB/MBDS Standard Library/Basic Operations/Logic and Bit Operations/AND  BitwiseMode=on  Inputs=1  UseBitMask=on  BitMask=bin2dec('00000010')  OutDataTypeStr=Inherit: Inherit via back propagation  PTC_MBDS_BlockVersion=5.41  PTC_BlockType=PTC_MBDS_AND
      settings: AttributesFormatString=bitwise  SourceProductName=PACCAR Technical Center MBDS Library
  AND2 : PTC_MBDS_LIB/MBDS Standard Library/Basic Operations/Logic and Bit Operations/AND  BitwiseMode=on  Inputs=1  UseBitMask=on  BitMask=bin2dec('00000100')  OutDataTypeStr=Inherit: Inherit via back propagation  PTC_MBDS_BlockVersion=5.41  PTC_BlockType=PTC_MBDS_AND
      settings: AttributesFormatString=bitwise  SourceProductName=PACCAR Technical Center MBDS Library
  AND3 : PTC_MBDS_LIB/MBDS Standard Library/Basic Operations/Logic and Bit Operations/AND  BitwiseMode=on  Inputs=1  UseBitMask=on  BitMask=bin2dec('00001000')  OutDataTypeStr=Inherit: Inherit via back propagation  PTC_MBDS_BlockVersion=5.41  PTC_BlockType=PTC_MBDS_AND
      settings: AttributesFormatString=bitwise  SourceProductName=PACCAR Technical Center MBDS Library
  AND4 : PTC_MBDS_LIB/MBDS Standard Library/Basic Operations/Logic and Bit Operations/AND  BitwiseMode=on  Inputs=1  UseBitMask=on  BitMask=bin2dec('00010000')  OutDataTypeStr=Inherit: Inherit via back propagation  PTC_MBDS_BlockVersion=5.41  PTC_BlockType=PTC_MBDS_AND
      settings: AttributesFormatString=bitwise  SourceProductName=PACCAR Technical Center MBDS Library
  AND5 : PTC_MBDS_LIB/MBDS Standard Library/Basic Operations/Logic and Bit Operations/AND  BitwiseMode=on  Inputs=1  UseBitMask=on  BitMask=bin2dec('00100000')  OutDataTypeStr=Inherit: Inherit via back propagation  PTC_MBDS_BlockVersion=5.41  PTC_BlockType=PTC_MBDS_AND
      settings: AttributesFormatString=bitwise  SourceProductName=PACCAR Technical Center MBDS Library
  Data Type Conversion : DataTypeConversion  OutDataTypeStr=uint8  SaturateOnIntegerOverflow=on
  Data Type Conversion{2..7} (6 alike) : DataTypeConversion  OutDataTypeStr=boolean  SaturateOnIntegerOverflow=on
  "Shift_Arithmetic " : ArithShift  BitShiftNumber=1
  Shift_Arithmetic 1 : ArithShift  BitShiftNumber=2
  Shift_Arithmetic 2 : ArithShift  BitShiftNumber=3
  Shift_Arithmetic 3 : ArithShift  BitShiftNumber=4
  Shift_Arithmetic 4 : ArithShift  BitShiftNumber=5
  TX_CAN4 : Subsystem
  Terminator{,1..9} (10 alike) : Terminator
  wires:
  AND1/1 -> "Shift_Arithmetic "/1
  AND2/1 -> Shift_Arithmetic 1/1
  Channel/1 -> Data Type Conversion/1
  Data Type Conversion/1 -> AND/1, AND1/1, AND5/1, AND4/1, AND3/1, AND2/1
  AND/1 -> Data Type Conversion2/1
  "Shift_Arithmetic "/1 -> Data Type Conversion3/1
  Shift_Arithmetic 1/1 -> Data Type Conversion4/1
  AND3/1 -> Shift_Arithmetic 2/1
  Shift_Arithmetic 2/1 -> Data Type Conversion5/1
  AND4/1 -> Shift_Arithmetic 3/1
  Shift_Arithmetic 3/1 -> Data Type Conversion6/1
  AND5/1 -> Shift_Arithmetic 4/1
  Shift_Arithmetic 4/1 -> Data Type Conversion7/1
  Data/1 -> Terminator9/1, Terminator5/1, TX_CAN4/2(Data), Terminator7/1, Terminator3/1, Terminator1/1
  Data Type Conversion2/1 -> Terminator/1
  Data Type Conversion3/1 -> Terminator2/1
  Data Type Conversion4/1 -> Terminator6/1
  Data Type Conversion5/1 -> TX_CAN4/1(Enable)
  Data Type Conversion6/1 -> Terminator4/1
  Data Type Conversion7/1 -> Terminator8/1

== system SUB_ECU_L4_MABX_HW_Interface_PTC_1571/CAN_Out_PTC_1571/CAN_TX_10ms/CAN_TX_EEC1_00 ==
  Channel : Inport  OutDataTypeStr=Enum: ENUM_CAN_TX_T
  Data : Inport  Port=2
  AND : PTC_MBDS_LIB/MBDS Standard Library/Basic Operations/Logic and Bit Operations/AND  BitwiseMode=on  Inputs=1  UseBitMask=on  BitMask=bin2dec('00000001')  OutDataTypeStr=Inherit: Inherit via back propagation  PTC_MBDS_BlockVersion=5.41  PTC_BlockType=PTC_MBDS_AND
      settings: AttributesFormatString=bitwise  SourceProductName=PACCAR Technical Center MBDS Library
  AND1 : PTC_MBDS_LIB/MBDS Standard Library/Basic Operations/Logic and Bit Operations/AND  BitwiseMode=on  Inputs=1  UseBitMask=on  BitMask=bin2dec('00000010')  OutDataTypeStr=Inherit: Inherit via back propagation  PTC_MBDS_BlockVersion=5.41  PTC_BlockType=PTC_MBDS_AND
      settings: AttributesFormatString=bitwise  SourceProductName=PACCAR Technical Center MBDS Library
  AND2 : PTC_MBDS_LIB/MBDS Standard Library/Basic Operations/Logic and Bit Operations/AND  BitwiseMode=on  Inputs=1  UseBitMask=on  BitMask=bin2dec('00000100')  OutDataTypeStr=Inherit: Inherit via back propagation  PTC_MBDS_BlockVersion=5.41  PTC_BlockType=PTC_MBDS_AND
      settings: AttributesFormatString=bitwise  SourceProductName=PACCAR Technical Center MBDS Library
  AND3 : PTC_MBDS_LIB/MBDS Standard Library/Basic Operations/Logic and Bit Operations/AND  BitwiseMode=on  Inputs=1  UseBitMask=on  BitMask=bin2dec('00001000')  OutDataTypeStr=Inherit: Inherit via back propagation  PTC_MBDS_BlockVersion=5.41  PTC_BlockType=PTC_MBDS_AND
      settings: AttributesFormatString=bitwise  SourceProductName=PACCAR Technical Center MBDS Library
  AND4 : PTC_MBDS_LIB/MBDS Standard Library/Basic Operations/Logic and Bit Operations/AND  BitwiseMode=on  Inputs=1  UseBitMask=on  BitMask=bin2dec('00010000')  OutDataTypeStr=Inherit: Inherit via back propagation  PTC_MBDS_BlockVersion=5.41  PTC_BlockType=PTC_MBDS_AND
      settings: AttributesFormatString=bitwise  SourceProductName=PACCAR Technical Center MBDS Library
  AND5 : PTC_MBDS_LIB/MBDS Standard Library/Basic Operations/Logic and Bit Operations/AND  BitwiseMode=on  Inputs=1  UseBitMask=on  BitMask=bin2dec('00100000')  OutDataTypeStr=Inherit: Inherit via back propagation  PTC_MBDS_BlockVersion=5.41  PTC_BlockType=PTC_MBDS_AND
      settings: AttributesFormatString=bitwise  SourceProductName=PACCAR Technical Center MBDS Library
  Data Type Conversion : DataTypeConversion  OutDataTypeStr=uint8  SaturateOnIntegerOverflow=on
  Data Type Conversion{2..7} (6 alike) : DataTypeConversion  OutDataTypeStr=boolean  SaturateOnIntegerOverflow=on
  "Shift_Arithmetic " : ArithShift  BitShiftNumber=1
  Shift_Arithmetic 1 : ArithShift  BitShiftNumber=2
  Shift_Arithmetic 2 : ArithShift  BitShiftNumber=3
  Shift_Arithmetic 3 : ArithShift  BitShiftNumber=4
  Shift_Arithmetic 4 : ArithShift  BitShiftNumber=5
  TX_CAN4 : Subsystem
  TX_CAN5 : Subsystem
  Terminator{,1..3,6..9} (8 alike) : Terminator
  wires:
  Data Type Conversion7/1 -> Terminator8/1
  Data Type Conversion6/1 -> TX_CAN5/1(Enable)
  Data Type Conversion5/1 -> TX_CAN4/1(Enable)
  Data Type Conversion4/1 -> Terminator6/1
  Data Type Conversion3/1 -> Terminator2/1
  Data Type Conversion2/1 -> Terminator/1
  Data/1 -> Terminator1/1, Terminator3/1, Terminator7/1, TX_CAN4/2(Data), TX_CAN5/2(Data), Terminator9/1
  Shift_Arithmetic 4/1 -> Data Type Conversion7/1
  AND5/1 -> Shift_Arithmetic 4/1
  Shift_Arithmetic 3/1 -> Data Type Conversion6/1
  AND4/1 -> Shift_Arithmetic 3/1
  Shift_Arithmetic 2/1 -> Data Type Conversion5/1
  AND3/1 -> Shift_Arithmetic 2/1
  Shift_Arithmetic 1/1 -> Data Type Conversion4/1
  "Shift_Arithmetic "/1 -> Data Type Conversion3/1
  AND/1 -> Data Type Conversion2/1
  Data Type Conversion/1 -> AND2/1, AND3/1, AND4/1, AND5/1, AND1/1, AND/1
  Channel/1 -> Data Type Conversion/1
  AND2/1 -> Shift_Arithmetic 1/1
  AND1/1 -> "Shift_Arithmetic "/1

== system SUB_ECU_L4_MABX_HW_Interface_PTC_1571/CAN_Out_PTC_1571/CAN_TX_10ms/CAN_TX_PROPB_REAX_1_E4 ==
  enable : Inport
  RawData : Inport  Port=2  OutDataTypeStr=uint8
  Bus Selector : BusSelector  OutputSignals=INPUTS.CAN.CANenable.EnablePropB_ReAX_CAN1,INPUTS.CAN.CANenable.EnablePropB_ReAX_CAN2
  Data Type Conversion1 : DataTypeConversion  SaturateOnIntegerOverflow=on
  TX_CAN1 : Subsystem
  TX_CAN2 : Subsystem
  wires:
  Bus Selector/2 -> TX_CAN2/1(Enable)  "<EnablePropB_ReAX_CAN2>"
  Bus Selector/1 -> TX_CAN1/1(Enable)  "<EnablePropB_ReAX_CAN1>"
  Data Type Conversion1/1 -> TX_CAN2/2(RawData), TX_CAN1/2(RawData)
  RawData/1 -> Data Type Conversion1/1
  enable/1 -> Bus Selector/1

== system SUB_ECU_L4_MABX_HW_Interface_PTC_1571/CAN_Out_PTC_1571/CAN_TX_10ms/CAN_TX_VDC2_0B ==
  Channel : Inport  OutDataTypeStr=Enum: ENUM_CAN_TX_T
  Data : Inport  Port=2
  AND : PTC_MBDS_LIB/MBDS Standard Library/Basic Operations/Logic and Bit Operations/AND  BitwiseMode=on  Inputs=1  UseBitMask=on  BitMask=bin2dec('00000001')  OutDataTypeStr=Inherit: Inherit via back propagation  PTC_MBDS_BlockVersion=5.41  PTC_BlockType=PTC_MBDS_AND
      settings: AttributesFormatString=bitwise  SourceProductName=PACCAR Technical Center MBDS Library
  AND1 : PTC_MBDS_LIB/MBDS Standard Library/Basic Operations/Logic and Bit Operations/AND  BitwiseMode=on  Inputs=1  UseBitMask=on  BitMask=bin2dec('00000010')  OutDataTypeStr=Inherit: Inherit via back propagation  PTC_MBDS_BlockVersion=5.41  PTC_BlockType=PTC_MBDS_AND
      settings: AttributesFormatString=bitwise  SourceProductName=PACCAR Technical Center MBDS Library
  AND2 : PTC_MBDS_LIB/MBDS Standard Library/Basic Operations/Logic and Bit Operations/AND  BitwiseMode=on  Inputs=1  UseBitMask=on  BitMask=bin2dec('00000100')  OutDataTypeStr=Inherit: Inherit via back propagation  PTC_MBDS_BlockVersion=5.41  PTC_BlockType=PTC_MBDS_AND
      settings: AttributesFormatString=bitwise  SourceProductName=PACCAR Technical Center MBDS Library
  AND3 : PTC_MBDS_LIB/MBDS Standard Library/Basic Operations/Logic and Bit Operations/AND  BitwiseMode=on  Inputs=1  UseBitMask=on  BitMask=bin2dec('00001000')  OutDataTypeStr=Inherit: Inherit via back propagation  PTC_MBDS_BlockVersion=5.41  PTC_BlockType=PTC_MBDS_AND
      settings: AttributesFormatString=bitwise  SourceProductName=PACCAR Technical Center MBDS Library
  AND4 : PTC_MBDS_LIB/MBDS Standard Library/Basic Operations/Logic and Bit Operations/AND  BitwiseMode=on  Inputs=1  UseBitMask=on  BitMask=bin2dec('00010000')  OutDataTypeStr=Inherit: Inherit via back propagation  PTC_MBDS_BlockVersion=5.41  PTC_BlockType=PTC_MBDS_AND
      settings: AttributesFormatString=bitwise  SourceProductName=PACCAR Technical Center MBDS Library
  AND5 : PTC_MBDS_LIB/MBDS Standard Library/Basic Operations/Logic and Bit Operations/AND  BitwiseMode=on  Inputs=1  UseBitMask=on  BitMask=bin2dec('00100000')  OutDataTypeStr=Inherit: Inherit via back propagation  PTC_MBDS_BlockVersion=5.41  PTC_BlockType=PTC_MBDS_AND
      settings: AttributesFormatString=bitwise  SourceProductName=PACCAR Technical Center MBDS Library
  Data Type Conversion : DataTypeConversion  OutDataTypeStr=uint8  SaturateOnIntegerOverflow=on
  Data Type Conversion{1,3..7} (6 alike) : DataTypeConversion  OutDataTypeStr=boolean  SaturateOnIntegerOverflow=on
  "Shift_Arithmetic " : ArithShift  BitShiftNumber=1
  Shift_Arithmetic 1 : ArithShift  BitShiftNumber=2
  Shift_Arithmetic 2 : ArithShift  BitShiftNumber=3
  Shift_Arithmetic 3 : ArithShift  BitShiftNumber=4
  Shift_Arithmetic 4 : ArithShift  BitShiftNumber=5
  TX_CAN5 : Subsystem
  Terminator{,1..9} (10 alike) : Terminator
  wires:
  Data Type Conversion7/1 -> Terminator8/1
  Data Type Conversion6/1 -> TX_CAN5/1(Enable)
  Data Type Conversion5/1 -> Terminator6/1
  Data Type Conversion4/1 -> Terminator4/1
  Data Type Conversion3/1 -> Terminator2/1
  Data Type Conversion1/1 -> Terminator/1
  Data/1 -> Terminator1/1, Terminator3/1, Terminator5/1, Terminator7/1, Terminator9/1, TX_CAN5/2(Data)
  Shift_Arithmetic 4/1 -> Data Type Conversion7/1
  AND5/1 -> Shift_Arithmetic 4/1
  Shift_Arithmetic 3/1 -> Data Type Conversion6/1
  AND4/1 -> Shift_Arithmetic 3/1
  Shift_Arithmetic 2/1 -> Data Type Conversion5/1
  AND3/1 -> Shift_Arithmetic 2/1
  Shift_Arithmetic 1/1 -> Data Type Conversion4/1
  "Shift_Arithmetic "/1 -> Data Type Conversion3/1
  AND/1 -> Data Type Conversion1/1
  Data Type Conversion/1 -> AND2/1, AND3/1, AND4/1, AND5/1, AND1/1, AND/1
  Channel/1 -> Data Type Conversion/1
  AND2/1 -> Shift_Arithmetic 1/1
  AND1/1 -> "Shift_Arithmetic "/1

== system SUB_ECU_L4_MABX_HW_Interface_PTC_1571/CAN_Out_PTC_1571/CAN_TX_10ms/Encode_PROPB_REAX_1 ==
  In1 : Inport
  Bus Selector : BusSelector  OutputSignals=10msTask.SteeringControl.DesSteeringAngle
  Bus Selector1 : BusSelector  OutputSignals=INPUTS.DIO_Bus.OperatorEnableSwitch
  CAN_ID_PropB_REAX_1_E4 : Subsystem
  Data Type Conversion : DataTypeConversion  OutDataTypeStr=uint8
  Encode_PROPB_REAX_1 : Subsystem
  PropB_REAX_1_E4_CommandFromExternalController : Subsystem
  PropB_REAX_1_E4_DesiredOperatingMode : Subsystem
  PropB_REAX_1_E4_MessageCounter : Subsystem
  Out1 : Outport
  wires:
  Data Type Conversion/1 -> PropB_REAX_1_E4_CommandFromExternalController/2(operatorEnable), PropB_REAX_1_E4_DesiredOperatingMode/1(OperatorEnable)
  Bus Selector/1 -> PropB_REAX_1_E4_CommandFromExternalController/1(DesiredSteeringAngle)  "<DesSteeringAngle>"
  Bus Selector1/1 -> Data Type Conversion/1  "<OperatorEnableSwitch>"
  CAN_ID_PropB_REAX_1_E4/1(MessageID) -> Encode_PROPB_REAX_1/1(MessageID)
  PropB_REAX_1_E4_DesiredOperatingMode/1(DesiredOperatingMode) -> Encode_PROPB_REAX_1/2(DesiredOperatingMode)
  Encode_PROPB_REAX_1/1(Data) -> Out1/1
  PropB_REAX_1_E4_MessageCounter/1(MessageCounter) -> Encode_PROPB_REAX_1/4(MessageCounter)
  PropB_REAX_1_E4_CommandFromExternalController/1(CommandFromExternalController) -> Encode_PROPB_REAX_1/3(CommandFromExternalController)
  In1/1 -> Bus Selector1/1, Bus Selector/1

== system SUB_ECU_L4_MABX_HW_Interface_PTC_1571/CAN_Out_PTC_1571/CAN_TX_20ms/CAN_TX_PROPB_XBR_B3 ==
  Channel : Inport
  Data : Inport  Port=2
  OperatorEnable : Inport  Port=3
  AND : PTC_MBDS_LIB/MBDS Standard Library/Basic Operations/Logic and Bit Operations/AND  BitwiseMode=on  Inputs=1  UseBitMask=on  BitMask=bin2dec('00000001')  OutDataTypeStr=Inherit: Inherit via back propagation  PTC_MBDS_BlockVersion=5.41  PTC_BlockType=PTC_MBDS_AND
      settings: AttributesFormatString=bitwise  SourceProductName=PACCAR Technical Center MBDS Library
  Bus Selector2 : BusSelector  OutputSignals=XBRPassThroughActive
  Compare To Constant : simulink/Logic and Bit Operations/Compare To Constant  relop===  const=ENUM_XBR_PASS_THROUGH_ACTIVE_T.ACTIVE  OutDataTypeStr=boolean
  Data Type Conversion : DataTypeConversion  OutDataTypeStr=uint8  SaturateOnIntegerOverflow=on
  Data Type Conversion2 : DataTypeConversion  OutDataTypeStr=boolean  SaturateOnIntegerOverflow=on
  Logical Operator : Logic  AllPortsSameDT=off  OutDataTypeStr=boolean
  Logical Operator1 : Logic  Operator=OR  AllPortsSameDT=off  OutDataTypeStr=boolean
  Logical Operator7 : Logic  AllPortsSameDT=off  OutDataTypeStr=boolean
  Logical Operator8 : Logic  Operator=NOT  AllPortsSameDT=off  OutDataTypeStr=boolean
  TX_CAN1 : Subsystem
  Terminator : Terminator
  Unit_Delay : UnitDelay  InitialCondition=false  SampleTime=-1
      settings: AttributesFormatString=IC: %<vinit>
  wires:
  Compare To Constant/1 -> Terminator/1
  OperatorEnable/1 -> Unit_Delay/1, Logical Operator8/1, Logical Operator1/2
  Unit_Delay/1 -> Logical Operator7/1
  Logical Operator8/1 -> Logical Operator7/2
  Logical Operator/1 -> TX_CAN1/1(Enable)
  Logical Operator1/1 -> Logical Operator/1
  Logical Operator7/1 -> Logical Operator1/1
  Data Type Conversion2/1 -> Logical Operator/2
  Data/1 -> Bus Selector2/1, TX_CAN1/2(Data)
  Channel/1 -> Data Type Conversion/1
  Data Type Conversion/1 -> AND/1
  AND/1 -> Data Type Conversion2/1
  Bus Selector2/1 -> Compare To Constant/1  "<XBRPassThroughActive>"
